simulink model "KF_Discrete"  (R2021b)
settings: Solver=VariableStepAuto  StartTime=0.0  StopTime=10  RelTol=1e-3
values from neighbouring files (symbols this model uses):
  sys2d = c2d(sys2,Ts)    [simConstants.m]
  Ts = 1e-3    (= 0.001)    [simConstants.m]
undefined symbols (not defined in the file or in its folder): Ld
libraries: simulink_extras x4
settings Model: Creator=logan  LastModifiedBy=logan

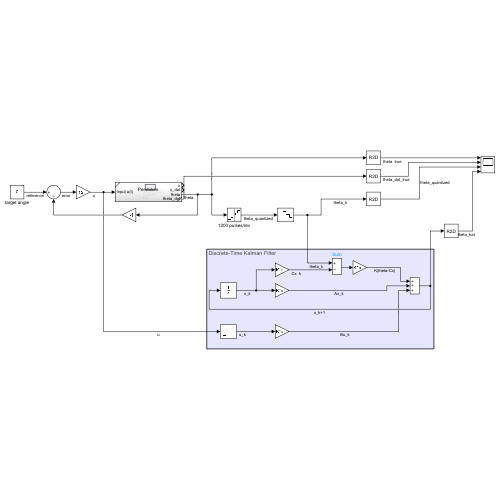
[thumbnail: Simulink's stored preview of the top-level diagram]
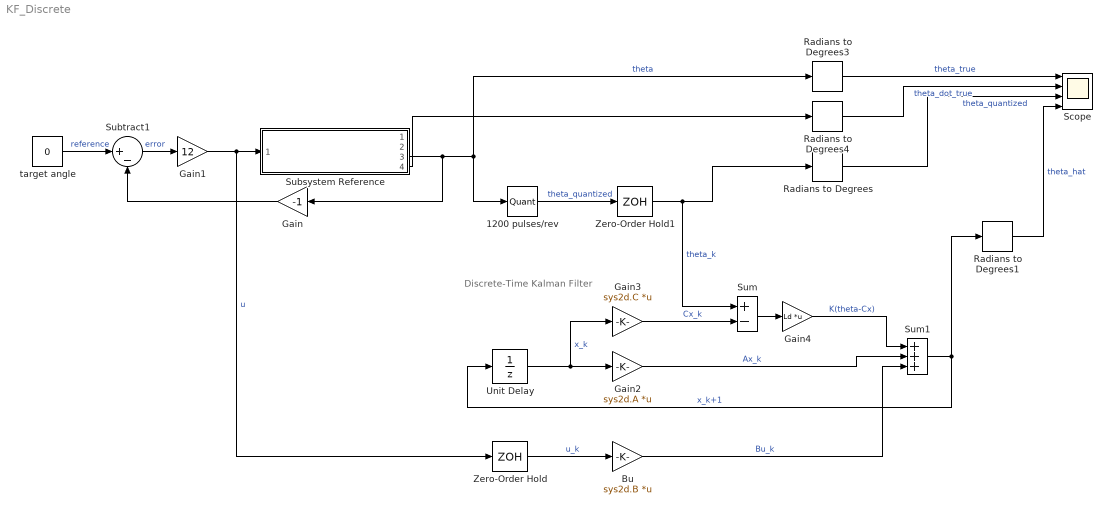
== system KF_Discrete ==
  note: Discrete-Time Kalman Filter
  1200 pulses/rev : Quantizer  QuantizationInterval=(2*pi)/1200
  Bu : Gain  Gain=sys2d.B  Multiplication=Matrix(K*u)
  Gain : Gain  Gain=-1
  Gain1 : Gain  Gain=12
  Gain2 : Gain  Gain=sys2d.A  Multiplication=Matrix(K*u)
  Gain3 : Gain  Gain=sys2d.C  Multiplication=Matrix(K*u)
  Gain4 : Gain  Gain=Ld  Multiplication=Matrix(K*u)
  Radians to Degrees{,1,3..4} (4 alike) : simulink_extras/Transformations/Radians to Degrees
  Scope : Scope  NumInputPorts=4
  Subsystem Reference : Subsystem  ReferencedSubsystem=Pendulum
  Subtract1 : Sum  Inputs=|+-
  Sum : Sum  Inputs=+-
  Sum1 : Sum  Inputs=+++
  Unit Delay : UnitDelay  SampleTime=Ts  HasFrameUpgradeWarning=on
  Zero-Order Hold : ZeroOrderHold  SampleTime=Ts
  Zero-Order Hold1 : ZeroOrderHold  SampleTime=Ts
  target angle : Constant  Value=0  OutDataTypeStr=Inherit: Inherit via back propagation
  wires:
  Subsystem Reference/3 -> Gain/1, Radians to Degrees3/1, 1200 pulses/rev/1  "theta"
  1200 pulses/rev/1 -> Zero-Order Hold1/1  "theta_quantized"
  Gain/1 -> Subtract1/2
  target angle/1 -> Subtract1/1  "reference"
  Gain1/1 -> Zero-Order Hold/1, Subsystem Reference/1  "u"
  Subtract1/1 -> Gain1/1  "error"
  Radians to Degrees/1 -> Scope/3  "theta_quantized"
  Radians to Degrees1/1 -> Scope/4  "theta_hat"
  Radians to Degrees3/1 -> Scope/1  "theta_true"
  Subsystem Reference/4 -> Radians to Degrees4/1
  Radians to Degrees4/1 -> Scope/2  "theta_dot_true"
  Zero-Order Hold1/1 -> Radians to Degrees/1, Sum/1  "theta_k"
  Sum1/1 -> Unit Delay/1, Radians to Degrees1/1  "x_k+1"
  Unit Delay/1 -> Gain3/1, Gain2/1  "x_k"
  Bu/1 -> Sum1/3  "Bu_k"
  Gain2/1 -> Sum1/2  "Ax_k"
  Zero-Order Hold/1 -> Bu/1  "u_k"
  Gain3/1 -> Sum/2  "Cx_k"
  Sum/1 -> Gain4/1
  Gain4/1 -> Sum1/1  "K(theta-Cx)"
